simulink library "PLL_three_phase_lib_2011"  (Simulink 7.8)
settings: Solver=ode45  StartTime=0.0  StopTime=10.0  RelTol=1e-3
values from neighbouring files (symbols this model uses):
  f = 60    [global_parameters.m]
  PLL_time_step = Ts    (= 8e-05)    [global_parameters.m]
undefined symbols (not defined in the file or in its folder): DiscIntNeverNeededParam
libraries: simulink x4, abc_dq_lib_2011 x1
settings Model: Creator=CH24070  LastModifiedBy=CH24070

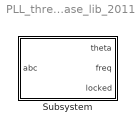
== system PLL_three_phase_lib_2011 ==
  Subsystem : Subsystem  mask{PLL_Kp=20*30, PLL_Ki=26*30, PLL_freq_range=0.25, PLL_lock_window=0.1}
      mask prompts: PLL_Kp "Proportional Gain"; PLL_Ki "Integral Gain"; PLL_freq_range "PLL Frequency Range"; PLL_lock_window "PLL Lock Window"

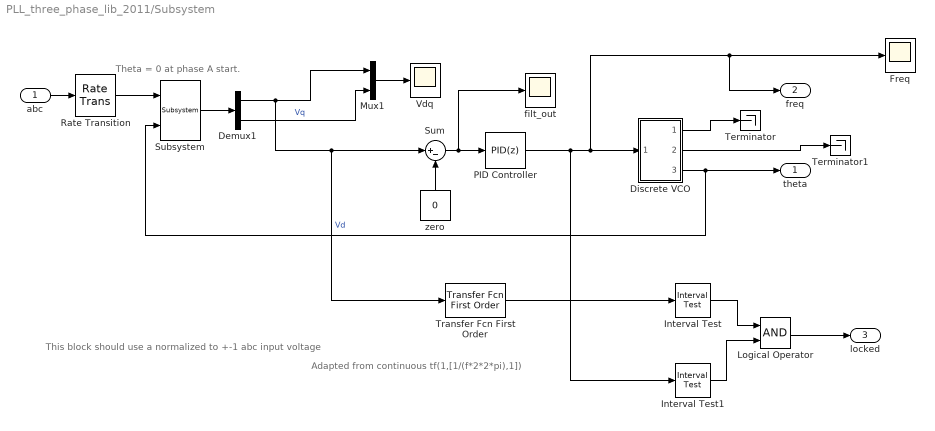
== system PLL_three_phase_lib_2011/Subsystem ==
  note: Adapted from continuous
      | tf(1,[1/(f*2*2*pi),1])
  note: This block should use a normalized to +-1 abc input voltage
  note: Theta = 0 at phase A start.
  abc : Inport  PortDimensions=3
  Demux1 : Demux  Outputs=2
  Discrete VCO : Subsystem
  Freq : Scope
      settings: TimeRange=0.1  YMin=368.5  YMax=378  SaveName=ScopeData2
  Interval Test : simulink/Logic and Bit Operations/Interval Test  IntervalClosedRight=on  uplimit=PLL_lock_window  IntervalClosedLeft=on  lowlimit=-PLL_lock_window  OutDataTypeStr=boolean
  Interval Test1 : simulink/Logic and Bit Operations/Interval Test  IntervalClosedRight=on  uplimit=2*pi*f*(1+PLL_freq_range)  IntervalClosedLeft=on  lowlimit=2*pi*f*(1-PLL_freq_range)  OutDataTypeStr=boolean
  Logical Operator : Logic  AllPortsSameDT=off  OutDataTypeStr=boolean
  Mux1 : Mux  Inputs=2
  PID Controller : simulink/Continuous/PID Controller  Controller=PID  TimeDomain=Discrete-time  SampleTime=PLL_time_step  IntegratorMethod=Forward Euler  FilterMethod=Forward Euler  Form=Parallel  P=PLL_Kp  I=PLL_Ki  D=0  N=100  InitialConditionSource=internal  InitialConditionForIntegrator=2*pi*f  InitialConditionForFilter=0  ExternalReset=none  ZeroCross=off  LimitOutput=on  UpperSaturationLimit=2*pi*(f*(1+PLL_freq_range))  LowerSaturationLimit=2*pi*(f*(1-PLL_freq_range))  LinearizeAsGain=on  AntiWindupMode=clamping  Kb=1  TrackingMode=off  Kt=1  PParamMin=[]  PParamMax=[]  IParamMin=[]  IParamMax=[]  DParamMin=[]  DParamMax=[]  NParamMin=[]  NParamMax=[]  KbParamMin=[]  KbParamMax=[]  KtParamMin=[]  KtParamMax=[]  POutMin=[]  POutMax=[]  IOutMin=[]  IOutMax=[]  DOutMin=[]  DOutMax=[]  NOutMin=[]  NOutMax=[]  KbOutMin=[]  KbOutMax=[]  KtOutMin=[]  KtOutMax=[]  IntegratorOutMin=[]  IntegratorOutMax=[]  FilterOutMin=[]  FilterOutMax=[]  SumOutMin=[]  SumOutMax=[]  SumI1OutMin=[]  SumI1OutMax=[]  SumI2OutMin=[]  SumI2OutMax=[]  SumI3OutMin=[]  SumI3OutMax=[]  SumDOutMin=[]  SumDOutMax=[]  SaturationOutMin=[]  SaturationOutMax=[]  IntegratorContinuousStateAttributes=''  IntegratorStateMustResolveToSignalObject=off  IntegratorRTWStateStorageClass=Auto  FilterContinuousStateAttributes=''  FilterStateMustResolveToSignalObject=off  FilterRTWStateStorageClass=Auto
  Rate Transition : RateTransition  OutPortSampleTime=PLL_time_step
  Subsystem : abc_dq_lib_2011/Subsystem
  Sum : Sum  Inputs=|+-
  Terminator : Terminator
  Terminator1 : Terminator
  Transfer Fcn First Order : simulink/Discrete/Transfer Fcn First Order  PoleZ=0.9274  ICPrevOutput=0.0  DoSatur=off
  Vdq : Scope
      settings: TimeRange=2  YMin=-1.75  YMax=1.75
  filt_out : Scope
      settings: TimeRange=2  YMin=-0.7  YMax=0.15  SaveName=ScopeData3
  zero : Constant  Value=0
  theta : Outport
  freq : Outport  Port=2
  locked : Outport  Port=3
  wires:
  Sum/1 -> filt_out/1, PID Controller/1
  Transfer Fcn First Order/1 -> Interval Test/1
  Discrete VCO/2(Sin) -> Terminator1/1
  PID Controller/1 -> Interval Test1/1, Discrete VCO/1(In1), freq/1, Freq/1
  Discrete VCO/1(Cos) -> Terminator/1
  Subsystem/1 -> Demux1/1
  Mux1/1 -> Vdq/1
  abc/1 -> Rate Transition/1
  Interval Test1/1 -> Logical Operator/2
  Demux1/2 -> Mux1/2  "Vq"
  Interval Test/1 -> Logical Operator/1
  zero/1 -> Sum/2
  Rate Transition/1 -> Subsystem/1
  Logical Operator/1 -> locked/1
  Discrete VCO/3(theta) -> Subsystem/2, theta/1
  Demux1/1 -> Transfer Fcn First Order/1, Sum/1, Mux1/1  "Vd"

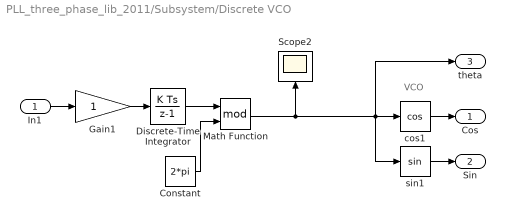
== system PLL_three_phase_lib_2011/Subsystem/Discrete VCO ==
  note: VCO
  In1 : Inport
  Constant : Constant  Value=2*pi
  Discrete-Time Integrator : DiscreteIntegrator  InitialConditionMode=State only (most efficient)  SampleTime=PLL_time_step  ICPrevOutput=DiscIntNeverNeededParam  ICPrevScaledInput=DiscIntNeverNeededParam
  Gain1 : Gain  OutDataTypeStr=double
  Math Function : Math  Operator=mod  SaturateOnIntegerOverflow=on
  Scope2 : Scope
      settings: TimeRange=0.1  YMin=0  YMax=70000
  cos1 : Trigonometry  Operator=cos
  sin1 : Trigonometry
  Cos : Outport
  Sin : Outport  Port=2
  theta : Outport  Port=3
  wires:
  In1/1 -> Gain1/1
  cos1/1 -> Cos/1
  sin1/1 -> Sin/1
  Constant/1 -> Math Function/2
  Gain1/1 -> Discrete-Time Integrator/1
  Discrete-Time Integrator/1 -> Math Function/1
  Math Function/1 -> Scope2/1, theta/1, cos1/1, sin1/1
